simulink model "ResearchPaper4Fig9"  (R2015b)
settings: Solver=VariableStepAuto  StartTime=0.0  StopTime=10.0  RelTol=1e-3
libraries: xbsIndex_r4 x942, commfilt2 x1, commrandsrc3 x1, commdigbbndam3 x1
(part 2 of 6)

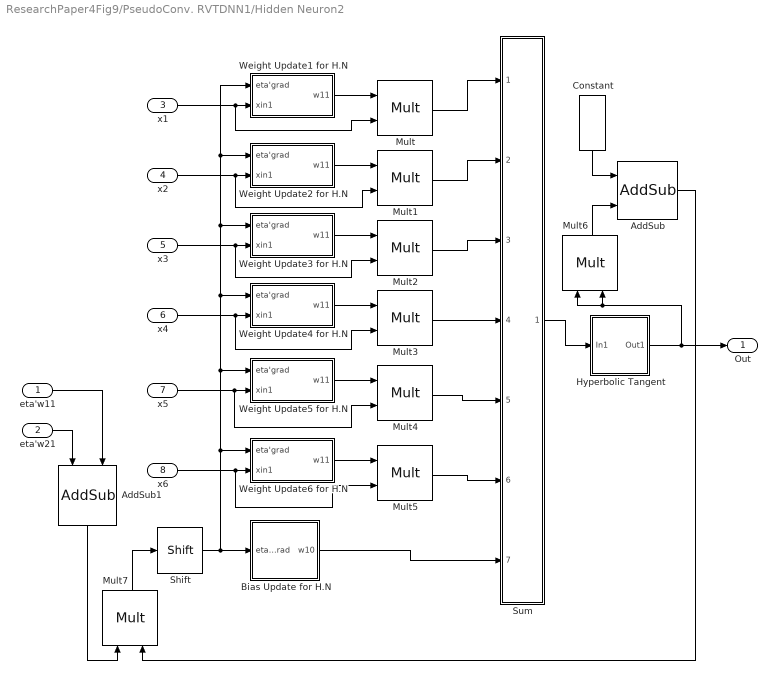
== system ResearchPaper4Fig9/PseudoConv. RVTDNN1/Hidden Neuron2 ==
  eta'w11 : Inport
  eta'w21 : Inport  Port=2
  x1 : Inport  Port=3
  x2 : Inport  Port=4
  x3 : Inport  Port=5
  x4 : Inport  Port=6
  x5 : Inport  Port=7
  x6 : Inport  Port=8
  AddSub : xbsIndex_r4/AddSub  mode=Subtraction  use_carryin=off  use_carryout=off  en=off  latency=0  precision=Full  arith_type=Unsigned  n_bits=16  bin_pt=14  quantization=Truncate  overflow=Wrap  use_behavioral_HDL=off  hw_selection=Fabric  pipelined=off  dbl_ovrd=off  block_type=addsub
  AddSub1 : xbsIndex_r4/AddSub  mode=Addition  use_carryin=off  use_carryout=off  en=off  latency=0  precision=Full  arith_type=Unsigned  n_bits=16  bin_pt=14  quantization=Truncate  overflow=Wrap  use_behavioral_HDL=off  hw_selection=Fabric  pipelined=off  dbl_ovrd=off  block_type=addsub
  Bias Update for H.N : Subsystem
  Constant : xbsIndex_r4/Constant  const=1.0  gui_display_data_type=Fixed-point  arith_type=Signed (2's comp)  n_bits=16  bin_pt=14  preci_type=Single  exp_width=8  frac_width=24  explicit_period=off  period=1  equ=P=C  opselect=C  inp2=PCIN>>17  opr=+  inp1=P  carry=CIN  dbl_ovrd=off  block_type=constant
  Hyperbolic Tangent : Subsystem
  Mult{,1..7} (8 alike) : xbsIndex_r4/Mult  precision=Full  arith_type="Signed  (2's comp)"  n_bits=16  bin_pt=14  quantization=Truncate  overflow=Wrap  en=off  latency=0  use_behavioral_HDL=off  opt=Speed  use_embedded=on  optimum_pipeline=off  pipeline=on  dbl_ovrd=off  use_rpm=on  placement_style=Triangular  block_type=mult
  Shift : xbsIndex_r4/Shift  shift_dir=Right  shift_bits=4  en=off  latency=0  precision=Full  arith_type="Signed  (2's comp)"  n_bits=16  bin_pt=14  quantization=Truncate  overflow=Wrap  dbl_ovrd=off  block_type=shift
  Sum : Subsystem
  Weight Update1 for H.N : Subsystem
  Weight Update2 for H.N : Subsystem
  Weight Update3 for H.N : Subsystem
  Weight Update4 for H.N : Subsystem
  Weight Update5 for H.N : Subsystem
  Weight Update6 for H.N : Subsystem
  Out : Outport
  wires:
  Mult7/1 -> Shift/1
  Constant/1 -> AddSub/1
  Shift/1 -> Weight Update6 for H.N/1(eta'grad), Weight Update5 for H.N/1(eta'grad), Weight Update4 for H.N/1(eta'grad), Weight Update3 for H.N/1(eta'grad), Weight Update2 for H.N/1(eta'grad), Weight Update1 for H.N/1(eta'grad), Bias Update for H.N/1(eta'grad)
  Mult6/1 -> AddSub/2
  eta'w11/1 -> AddSub1/2
  Hyperbolic Tangent/1(Out1) -> Out/1, Mult6/1, Mult6/2
  AddSub1/1 -> Mult7/1
  AddSub/1 -> Mult7/2
  eta'w21/1 -> AddSub1/1
  Weight Update5 for H.N/1(w11) -> Mult4/1
  x3/1 -> Weight Update3 for H.N/2(xin1), Mult2/2
  x5/1 -> Weight Update5 for H.N/2(xin1), Mult4/2
  Weight Update6 for H.N/1(w11) -> Mult5/1
  Weight Update4 for H.N/1(w11) -> Mult3/1
  x2/1 -> Weight Update2 for H.N/2(xin1), Mult1/2
  Weight Update1 for H.N/1(w11) -> Mult/1
  Weight Update2 for H.N/1(w11) -> Mult1/1
  Weight Update3 for H.N/1(w11) -> Mult2/1
  x1/1 -> Mult/2, Weight Update1 for H.N/2(xin1)
  x4/1 -> Weight Update4 for H.N/2(xin1), Mult3/2
  x6/1 -> Weight Update6 for H.N/2(xin1), Mult5/2
  Mult/1 -> Sum/1(In1)
  Mult1/1 -> Sum/2(In2)
  Mult2/1 -> Sum/3(In3)
  Mult3/1 -> Sum/4(In4)
  Mult4/1 -> Sum/5(In5)
  Mult5/1 -> Sum/6(In6)
  Bias Update for H.N/1(w10) -> Sum/7(In7)
  Sum/1(Out) -> Hyperbolic Tangent/1(In1)

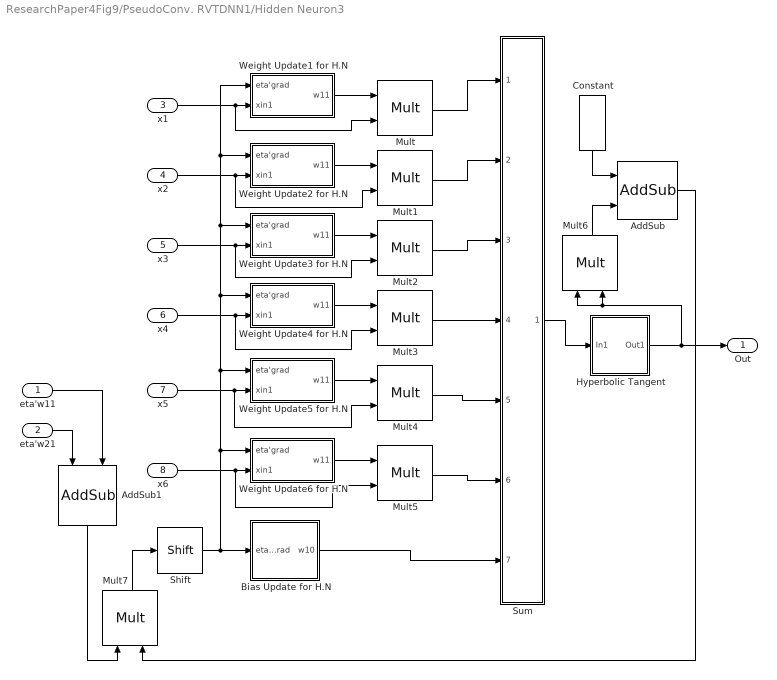
== system ResearchPaper4Fig9/PseudoConv. RVTDNN1/Hidden Neuron3 ==
  eta'w11 : Inport
  eta'w21 : Inport  Port=2
  x1 : Inport  Port=3
  x2 : Inport  Port=4
  x3 : Inport  Port=5
  x4 : Inport  Port=6
  x5 : Inport  Port=7
  x6 : Inport  Port=8
  AddSub : xbsIndex_r4/AddSub  mode=Subtraction  use_carryin=off  use_carryout=off  en=off  latency=0  precision=Full  arith_type=Unsigned  n_bits=16  bin_pt=14  quantization=Truncate  overflow=Wrap  use_behavioral_HDL=off  hw_selection=Fabric  pipelined=off  dbl_ovrd=off  block_type=addsub
  AddSub1 : xbsIndex_r4/AddSub  mode=Addition  use_carryin=off  use_carryout=off  en=off  latency=0  precision=Full  arith_type=Unsigned  n_bits=16  bin_pt=14  quantization=Truncate  overflow=Wrap  use_behavioral_HDL=off  hw_selection=Fabric  pipelined=off  dbl_ovrd=off  block_type=addsub
  Bias Update for H.N : Subsystem
  Constant : xbsIndex_r4/Constant  const=1.0  gui_display_data_type=Fixed-point  arith_type=Signed (2's comp)  n_bits=16  bin_pt=14  preci_type=Single  exp_width=8  frac_width=24  explicit_period=off  period=1  equ=P=C  opselect=C  inp2=PCIN>>17  opr=+  inp1=P  carry=CIN  dbl_ovrd=off  block_type=constant
  Hyperbolic Tangent : Subsystem
  Mult{,1..7} (8 alike) : xbsIndex_r4/Mult  precision=Full  arith_type="Signed  (2's comp)"  n_bits=16  bin_pt=14  quantization=Truncate  overflow=Wrap  en=off  latency=0  use_behavioral_HDL=off  opt=Speed  use_embedded=on  optimum_pipeline=off  pipeline=on  dbl_ovrd=off  use_rpm=on  placement_style=Triangular  block_type=mult
  Shift : xbsIndex_r4/Shift  shift_dir=Right  shift_bits=4  en=off  latency=0  precision=Full  arith_type="Signed  (2's comp)"  n_bits=16  bin_pt=14  quantization=Truncate  overflow=Wrap  dbl_ovrd=off  block_type=shift
  Sum : Subsystem
  Weight Update1 for H.N : Subsystem
  Weight Update2 for H.N : Subsystem
  Weight Update3 for H.N : Subsystem
  Weight Update4 for H.N : Subsystem
  Weight Update5 for H.N : Subsystem
  Weight Update6 for H.N : Subsystem
  Out : Outport
  wires:
  Mult7/1 -> Shift/1
  Constant/1 -> AddSub/1
  Shift/1 -> Weight Update6 for H.N/1(eta'grad), Weight Update5 for H.N/1(eta'grad), Weight Update4 for H.N/1(eta'grad), Weight Update3 for H.N/1(eta'grad), Weight Update2 for H.N/1(eta'grad), Weight Update1 for H.N/1(eta'grad), Bias Update for H.N/1(eta'grad)
  Mult6/1 -> AddSub/2
  eta'w11/1 -> AddSub1/2
  Hyperbolic Tangent/1(Out1) -> Out/1, Mult6/1, Mult6/2
  AddSub1/1 -> Mult7/1
  AddSub/1 -> Mult7/2
  eta'w21/1 -> AddSub1/1
  Weight Update5 for H.N/1(w11) -> Mult4/1
  x3/1 -> Weight Update3 for H.N/2(xin1), Mult2/2
  x5/1 -> Weight Update5 for H.N/2(xin1), Mult4/2
  Weight Update6 for H.N/1(w11) -> Mult5/1
  Weight Update4 for H.N/1(w11) -> Mult3/1
  x2/1 -> Weight Update2 for H.N/2(xin1), Mult1/2
  Weight Update1 for H.N/1(w11) -> Mult/1
  Weight Update2 for H.N/1(w11) -> Mult1/1
  Weight Update3 for H.N/1(w11) -> Mult2/1
  x1/1 -> Mult/2, Weight Update1 for H.N/2(xin1)
  x4/1 -> Weight Update4 for H.N/2(xin1), Mult3/2
  x6/1 -> Weight Update6 for H.N/2(xin1), Mult5/2
  Mult/1 -> Sum/1(In1)
  Mult1/1 -> Sum/2(In2)
  Mult2/1 -> Sum/3(In3)
  Mult3/1 -> Sum/4(In4)
  Mult4/1 -> Sum/5(In5)
  Mult5/1 -> Sum/6(In6)
  Bias Update for H.N/1(w10) -> Sum/7(In7)
  Sum/1(Out) -> Hyperbolic Tangent/1(In1)

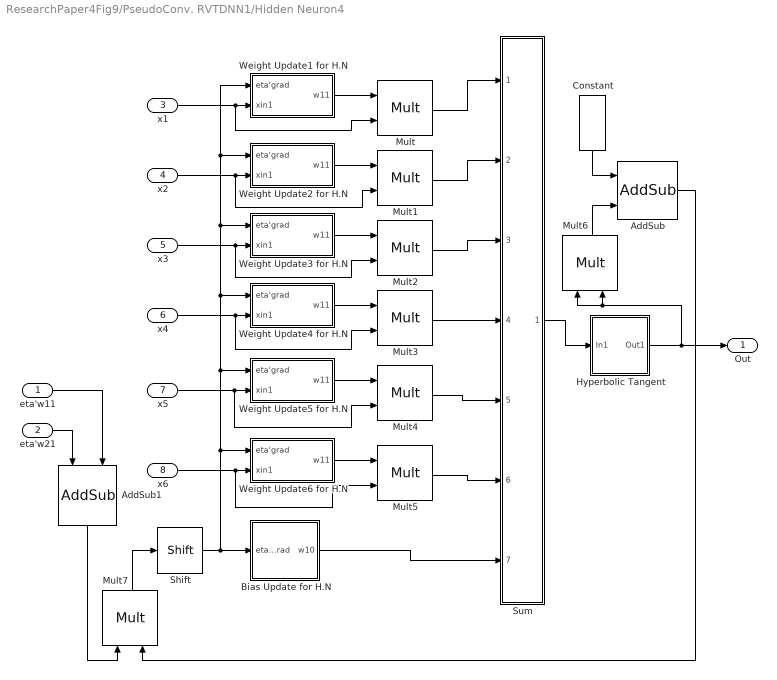
== system ResearchPaper4Fig9/PseudoConv. RVTDNN1/Hidden Neuron4 ==
  eta'w11 : Inport
  eta'w21 : Inport  Port=2
  x1 : Inport  Port=3
  x2 : Inport  Port=4
  x3 : Inport  Port=5
  x4 : Inport  Port=6
  x5 : Inport  Port=7
  x6 : Inport  Port=8
  AddSub : xbsIndex_r4/AddSub  mode=Subtraction  use_carryin=off  use_carryout=off  en=off  latency=0  precision=Full  arith_type=Unsigned  n_bits=16  bin_pt=14  quantization=Truncate  overflow=Wrap  use_behavioral_HDL=off  hw_selection=Fabric  pipelined=off  dbl_ovrd=off  block_type=addsub
  AddSub1 : xbsIndex_r4/AddSub  mode=Addition  use_carryin=off  use_carryout=off  en=off  latency=0  precision=Full  arith_type=Unsigned  n_bits=16  bin_pt=14  quantization=Truncate  overflow=Wrap  use_behavioral_HDL=off  hw_selection=Fabric  pipelined=off  dbl_ovrd=off  block_type=addsub
  Bias Update for H.N : Subsystem
  Constant : xbsIndex_r4/Constant  const=1.0  gui_display_data_type=Fixed-point  arith_type=Signed (2's comp)  n_bits=16  bin_pt=14  preci_type=Single  exp_width=8  frac_width=24  explicit_period=off  period=1  equ=P=C  opselect=C  inp2=PCIN>>17  opr=+  inp1=P  carry=CIN  dbl_ovrd=off  block_type=constant
  Hyperbolic Tangent : Subsystem
  Mult{,1..7} (8 alike) : xbsIndex_r4/Mult  precision=Full  arith_type="Signed  (2's comp)"  n_bits=16  bin_pt=14  quantization=Truncate  overflow=Wrap  en=off  latency=0  use_behavioral_HDL=off  opt=Speed  use_embedded=on  optimum_pipeline=off  pipeline=on  dbl_ovrd=off  use_rpm=on  placement_style=Triangular  block_type=mult
  Shift : xbsIndex_r4/Shift  shift_dir=Right  shift_bits=4  en=off  latency=0  precision=Full  arith_type="Signed  (2's comp)"  n_bits=16  bin_pt=14  quantization=Truncate  overflow=Wrap  dbl_ovrd=off  block_type=shift
  Sum : Subsystem
  Weight Update1 for H.N : Subsystem
  Weight Update2 for H.N : Subsystem
  Weight Update3 for H.N : Subsystem
  Weight Update4 for H.N : Subsystem
  Weight Update5 for H.N : Subsystem
  Weight Update6 for H.N : Subsystem
  Out : Outport
  wires:
  Mult7/1 -> Shift/1
  Constant/1 -> AddSub/1
  Shift/1 -> Weight Update6 for H.N/1(eta'grad), Weight Update5 for H.N/1(eta'grad), Weight Update4 for H.N/1(eta'grad), Weight Update3 for H.N/1(eta'grad), Weight Update2 for H.N/1(eta'grad), Weight Update1 for H.N/1(eta'grad), Bias Update for H.N/1(eta'grad)
  Mult6/1 -> AddSub/2
  eta'w11/1 -> AddSub1/2
  Hyperbolic Tangent/1(Out1) -> Out/1, Mult6/1, Mult6/2
  AddSub1/1 -> Mult7/1
  AddSub/1 -> Mult7/2
  eta'w21/1 -> AddSub1/1
  Weight Update5 for H.N/1(w11) -> Mult4/1
  x3/1 -> Weight Update3 for H.N/2(xin1), Mult2/2
  x5/1 -> Weight Update5 for H.N/2(xin1), Mult4/2
  Weight Update6 for H.N/1(w11) -> Mult5/1
  Weight Update4 for H.N/1(w11) -> Mult3/1
  x2/1 -> Weight Update2 for H.N/2(xin1), Mult1/2
  Weight Update1 for H.N/1(w11) -> Mult/1
  Weight Update2 for H.N/1(w11) -> Mult1/1
  Weight Update3 for H.N/1(w11) -> Mult2/1
  x1/1 -> Mult/2, Weight Update1 for H.N/2(xin1)
  x4/1 -> Weight Update4 for H.N/2(xin1), Mult3/2
  x6/1 -> Weight Update6 for H.N/2(xin1), Mult5/2
  Mult/1 -> Sum/1(In1)
  Mult1/1 -> Sum/2(In2)
  Mult2/1 -> Sum/3(In3)
  Mult3/1 -> Sum/4(In4)
  Mult4/1 -> Sum/5(In5)
  Mult5/1 -> Sum/6(In6)
  Bias Update for H.N/1(w10) -> Sum/7(In7)
  Sum/1(Out) -> Hyperbolic Tangent/1(In1)

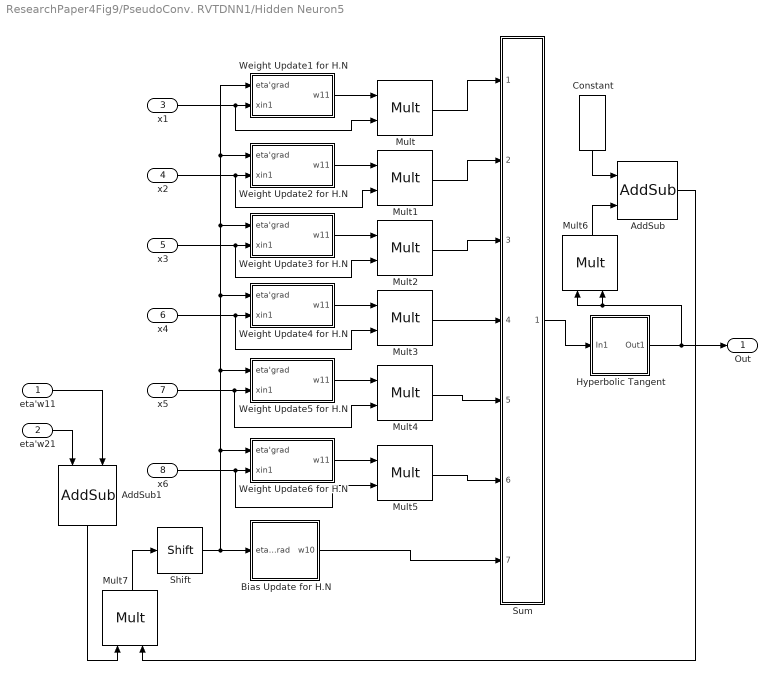
== system ResearchPaper4Fig9/PseudoConv. RVTDNN1/Hidden Neuron5 ==
  eta'w11 : Inport
  eta'w21 : Inport  Port=2
  x1 : Inport  Port=3
  x2 : Inport  Port=4
  x3 : Inport  Port=5
  x4 : Inport  Port=6
  x5 : Inport  Port=7
  x6 : Inport  Port=8
  AddSub : xbsIndex_r4/AddSub  mode=Subtraction  use_carryin=off  use_carryout=off  en=off  latency=0  precision=Full  arith_type=Unsigned  n_bits=16  bin_pt=14  quantization=Truncate  overflow=Wrap  use_behavioral_HDL=off  hw_selection=Fabric  pipelined=off  dbl_ovrd=off  block_type=addsub
  AddSub1 : xbsIndex_r4/AddSub  mode=Addition  use_carryin=off  use_carryout=off  en=off  latency=0  precision=Full  arith_type=Unsigned  n_bits=16  bin_pt=14  quantization=Truncate  overflow=Wrap  use_behavioral_HDL=off  hw_selection=Fabric  pipelined=off  dbl_ovrd=off  block_type=addsub
  Bias Update for H.N : Subsystem
  Constant : xbsIndex_r4/Constant  const=1.0  gui_display_data_type=Fixed-point  arith_type=Signed (2's comp)  n_bits=16  bin_pt=14  preci_type=Single  exp_width=8  frac_width=24  explicit_period=off  period=1  equ=P=C  opselect=C  inp2=PCIN>>17  opr=+  inp1=P  carry=CIN  dbl_ovrd=off  block_type=constant
  Hyperbolic Tangent : Subsystem
  Mult{,1..7} (8 alike) : xbsIndex_r4/Mult  precision=Full  arith_type="Signed  (2's comp)"  n_bits=16  bin_pt=14  quantization=Truncate  overflow=Wrap  en=off  latency=0  use_behavioral_HDL=off  opt=Speed  use_embedded=on  optimum_pipeline=off  pipeline=on  dbl_ovrd=off  use_rpm=on  placement_style=Triangular  block_type=mult
  Shift : xbsIndex_r4/Shift  shift_dir=Right  shift_bits=4  en=off  latency=0  precision=Full  arith_type="Signed  (2's comp)"  n_bits=16  bin_pt=14  quantization=Truncate  overflow=Wrap  dbl_ovrd=off  block_type=shift
  Sum : Subsystem
  Weight Update1 for H.N : Subsystem
  Weight Update2 for H.N : Subsystem
  Weight Update3 for H.N : Subsystem
  Weight Update4 for H.N : Subsystem
  Weight Update5 for H.N : Subsystem
  Weight Update6 for H.N : Subsystem
  Out : Outport
  wires:
  Mult7/1 -> Shift/1
  Constant/1 -> AddSub/1
  Shift/1 -> Weight Update6 for H.N/1(eta'grad), Weight Update5 for H.N/1(eta'grad), Weight Update4 for H.N/1(eta'grad), Weight Update3 for H.N/1(eta'grad), Weight Update2 for H.N/1(eta'grad), Weight Update1 for H.N/1(eta'grad), Bias Update for H.N/1(eta'grad)
  Mult6/1 -> AddSub/2
  eta'w11/1 -> AddSub1/2
  Hyperbolic Tangent/1(Out1) -> Out/1, Mult6/1, Mult6/2
  AddSub1/1 -> Mult7/1
  AddSub/1 -> Mult7/2
  eta'w21/1 -> AddSub1/1
  Weight Update5 for H.N/1(w11) -> Mult4/1
  x3/1 -> Weight Update3 for H.N/2(xin1), Mult2/2
  x5/1 -> Weight Update5 for H.N/2(xin1), Mult4/2
  Weight Update6 for H.N/1(w11) -> Mult5/1
  Weight Update4 for H.N/1(w11) -> Mult3/1
  x2/1 -> Weight Update2 for H.N/2(xin1), Mult1/2
  Weight Update1 for H.N/1(w11) -> Mult/1
  Weight Update2 for H.N/1(w11) -> Mult1/1
  Weight Update3 for H.N/1(w11) -> Mult2/1
  x1/1 -> Mult/2, Weight Update1 for H.N/2(xin1)
  x4/1 -> Weight Update4 for H.N/2(xin1), Mult3/2
  x6/1 -> Weight Update6 for H.N/2(xin1), Mult5/2
  Mult/1 -> Sum/1(In1)
  Mult1/1 -> Sum/2(In2)
  Mult2/1 -> Sum/3(In3)
  Mult3/1 -> Sum/4(In4)
  Mult4/1 -> Sum/5(In5)
  Mult5/1 -> Sum/6(In6)
  Bias Update for H.N/1(w10) -> Sum/7(In7)
  Sum/1(Out) -> Hyperbolic Tangent/1(In1)

== system ResearchPaper4Fig9/PseudoConv. RVTDNN1/Hidden Neuron6 ==
  eta'w11 : Inport
  eta'w21 : Inport  Port=2
  x1 : Inport  Port=3
  x2 : Inport  Port=4
  x3 : Inport  Port=5
  x4 : Inport  Port=6
  x5 : Inport  Port=7
  x6 : Inport  Port=8
  AddSub : xbsIndex_r4/AddSub  mode=Subtraction  use_carryin=off  use_carryout=off  en=off  latency=0  precision=Full  arith_type=Unsigned  n_bits=16  bin_pt=14  quantization=Truncate  overflow=Wrap  use_behavioral_HDL=off  hw_selection=Fabric  pipelined=off  dbl_ovrd=off  block_type=addsub
  AddSub1 : xbsIndex_r4/AddSub  mode=Addition  use_carryin=off  use_carryout=off  en=off  latency=0  precision=Full  arith_type=Unsigned  n_bits=16  bin_pt=14  quantization=Truncate  overflow=Wrap  use_behavioral_HDL=off  hw_selection=Fabric  pipelined=off  dbl_ovrd=off  block_type=addsub
  Bias Update for H.N : Subsystem
  Constant : xbsIndex_r4/Constant  const=1.0  gui_display_data_type=Fixed-point  arith_type=Signed (2's comp)  n_bits=16  bin_pt=14  preci_type=Single  exp_width=8  frac_width=24  explicit_period=off  period=1  equ=P=C  opselect=C  inp2=PCIN>>17  opr=+  inp1=P  carry=CIN  dbl_ovrd=off  block_type=constant
  Hyperbolic Tangent : Subsystem
  Mult{,1..7} (8 alike) : xbsIndex_r4/Mult  precision=Full  arith_type="Signed  (2's comp)"  n_bits=16  bin_pt=14  quantization=Truncate  overflow=Wrap  en=off  latency=0  use_behavioral_HDL=off  opt=Speed  use_embedded=on  optimum_pipeline=off  pipeline=on  dbl_ovrd=off  use_rpm=on  placement_style=Triangular  block_type=mult
  Shift : xbsIndex_r4/Shift  shift_dir=Right  shift_bits=4  en=off  latency=0  precision=Full  arith_type="Signed  (2's comp)"  n_bits=16  bin_pt=14  quantization=Truncate  overflow=Wrap  dbl_ovrd=off  block_type=shift
  Sum : Subsystem
  Weight Update1 for H.N : Subsystem
  Weight Update2 for H.N : Subsystem
  Weight Update3 for H.N : Subsystem
  Weight Update4 for H.N : Subsystem
  Weight Update5 for H.N : Subsystem
  Weight Update6 for H.N : Subsystem
  Out : Outport
  wires:
  Mult7/1 -> Shift/1
  Constant/1 -> AddSub/1
  Shift/1 -> Weight Update6 for H.N/1(eta'grad), Weight Update5 for H.N/1(eta'grad), Weight Update4 for H.N/1(eta'grad), Weight Update3 for H.N/1(eta'grad), Weight Update2 for H.N/1(eta'grad), Weight Update1 for H.N/1(eta'grad), Bias Update for H.N/1(eta'grad)
  Mult6/1 -> AddSub/2
  eta'w11/1 -> AddSub1/2
  Hyperbolic Tangent/1(Out1) -> Out/1, Mult6/1, Mult6/2
  AddSub1/1 -> Mult7/1
  AddSub/1 -> Mult7/2
  eta'w21/1 -> AddSub1/1
  Weight Update5 for H.N/1(w11) -> Mult4/1
  x3/1 -> Weight Update3 for H.N/2(xin1), Mult2/2
  x5/1 -> Weight Update5 for H.N/2(xin1), Mult4/2
  Weight Update6 for H.N/1(w11) -> Mult5/1
  Weight Update4 for H.N/1(w11) -> Mult3/1
  x2/1 -> Weight Update2 for H.N/2(xin1), Mult1/2
  Weight Update1 for H.N/1(w11) -> Mult/1
  Weight Update2 for H.N/1(w11) -> Mult1/1
  Weight Update3 for H.N/1(w11) -> Mult2/1
  x1/1 -> Mult/2, Weight Update1 for H.N/2(xin1)
  x4/1 -> Weight Update4 for H.N/2(xin1), Mult3/2
  x6/1 -> Weight Update6 for H.N/2(xin1), Mult5/2
  Mult/1 -> Sum/1(In1)
  Mult1/1 -> Sum/2(In2)
  Mult2/1 -> Sum/3(In3)
  Mult3/1 -> Sum/4(In4)
  Mult4/1 -> Sum/5(In5)
  Mult5/1 -> Sum/6(In6)
  Bias Update for H.N/1(w10) -> Sum/7(In7)
  Sum/1(Out) -> Hyperbolic Tangent/1(In1)

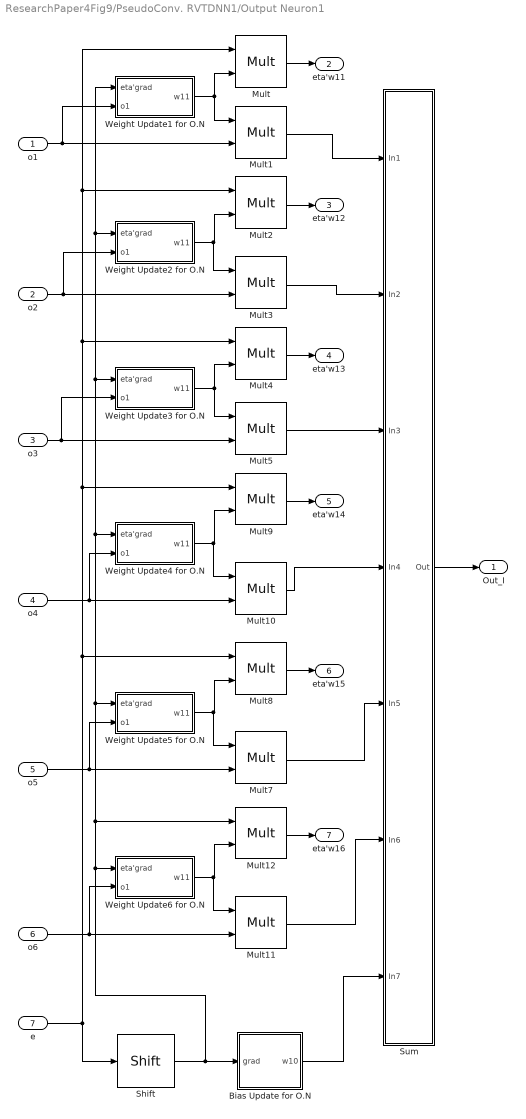
== system ResearchPaper4Fig9/PseudoConv. RVTDNN1/Output Neuron1 ==
  o1 : Inport
  o2 : Inport  Port=2
  o3 : Inport  Port=3
  o4 : Inport  Port=4
  o5 : Inport  Port=5
  o6 : Inport  Port=6
  e : Inport  Port=7
  Bias Update for O.N : Subsystem
  Mult{,1..5,7..12} (12 alike) : xbsIndex_r4/Mult  precision=Full  arith_type="Signed  (2's comp)"  n_bits=16  bin_pt=14  quantization=Truncate  overflow=Wrap  en=off  latency=0  use_behavioral_HDL=off  opt=Speed  use_embedded=on  optimum_pipeline=off  pipeline=on  dbl_ovrd=off  use_rpm=on  placement_style=Triangular  block_type=mult
  Shift : xbsIndex_r4/Shift  shift_dir=Right  shift_bits=4  en=off  latency=0  precision=Full  arith_type="Signed  (2's comp)"  n_bits=16  bin_pt=14  quantization=Truncate  overflow=Wrap  dbl_ovrd=off  block_type=shift
  Sum : Subsystem
  Weight Update1 for O.N : Subsystem
  Weight Update2 for O.N : Subsystem
  Weight Update3 for O.N : Subsystem
  Weight Update4 for O.N : Subsystem
  Weight Update5 for O.N : Subsystem
  Weight Update6 for O.N : Subsystem
  Out_I : Outport
  eta'w11 : Outport  Port=2
  eta'w12 : Outport  Port=3
  eta'w13 : Outport  Port=4
  eta'w14 : Outport  Port=5
  eta'w15 : Outport  Port=6
  eta'w16 : Outport  Port=7
  wires:
  o3/1 -> Weight Update3 for O.N/2(o1), Mult5/2
  o2/1 -> Weight Update2 for O.N/2(o1), Mult3/2
  o1/1 -> Weight Update1 for O.N/2(o1), Mult1/2
  o4/1 -> Weight Update4 for O.N/2(o1), Mult10/2
  Weight Update1 for O.N/1(w11) -> Mult1/1, Mult/2
  Weight Update2 for O.N/1(w11) -> Mult3/1, Mult2/2
  Weight Update3 for O.N/1(w11) -> Mult5/1, Mult4/2
  Weight Update4 for O.N/1(w11) -> Mult10/1, Mult9/2
  Mult/1 -> eta'w11/1
  Mult2/1 -> eta'w12/1
  Mult4/1 -> eta'w13/1
  Mult9/1 -> eta'w14/1
  Mult3/1 -> Sum/2(In2)
  Shift/1 -> Weight Update6 for O.N/1(eta'grad), Mult12/1, Weight Update5 for O.N/1(eta'grad), Weight Update4 for O.N/1(eta'grad), Weight Update3 for O.N/1(eta'grad), Weight Update2 for O.N/1(eta'grad), Weight Update1 for O.N/1(eta'grad), Bias Update for O.N/1(grad)
  e/1 -> Shift/1, Mult8/1, Mult4/1, Mult2/1, Mult/1, Mult9/1
  Sum/1(Out) -> Out_I/1
  o5/1 -> Weight Update5 for O.N/2(o1), Mult7/2
  Weight Update5 for O.N/1(w11) -> Mult7/1, Mult8/2
  Mult8/1 -> eta'w15/1
  o6/1 -> Weight Update6 for O.N/2(o1), Mult11/2
  Weight Update6 for O.N/1(w11) -> Mult11/1, Mult12/2
  Mult12/1 -> eta'w16/1
  Mult1/1 -> Sum/1(In1)
  Mult5/1 -> Sum/3(In3)
  Mult10/1 -> Sum/4(In4)
  Mult7/1 -> Sum/5(In5)
  Mult11/1 -> Sum/6(In6)
  Bias Update for O.N/1(w10) -> Sum/7(In7)

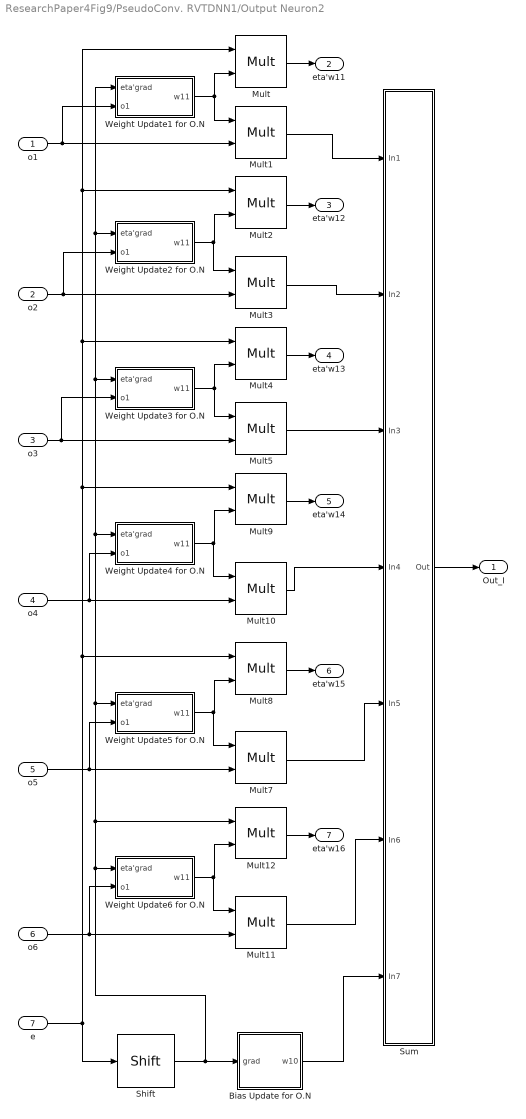
== system ResearchPaper4Fig9/PseudoConv. RVTDNN1/Output Neuron2 ==
  o1 : Inport
  o2 : Inport  Port=2
  o3 : Inport  Port=3
  o4 : Inport  Port=4
  o5 : Inport  Port=5
  o6 : Inport  Port=6
  e : Inport  Port=7
  Bias Update for O.N : Subsystem
  Mult{,1..5,7..12} (12 alike) : xbsIndex_r4/Mult  precision=Full  arith_type="Signed  (2's comp)"  n_bits=16  bin_pt=14  quantization=Truncate  overflow=Wrap  en=off  latency=0  use_behavioral_HDL=off  opt=Speed  use_embedded=on  optimum_pipeline=off  pipeline=on  dbl_ovrd=off  use_rpm=on  placement_style=Triangular  block_type=mult
  Shift : xbsIndex_r4/Shift  shift_dir=Right  shift_bits=4  en=off  latency=0  precision=Full  arith_type="Signed  (2's comp)"  n_bits=16  bin_pt=14  quantization=Truncate  overflow=Wrap  dbl_ovrd=off  block_type=shift
  Sum : Subsystem
  Weight Update1 for O.N : Subsystem
  Weight Update2 for O.N : Subsystem
  Weight Update3 for O.N : Subsystem
  Weight Update4 for O.N : Subsystem
  Weight Update5 for O.N : Subsystem
  Weight Update6 for O.N : Subsystem
  Out_I : Outport
  eta'w11 : Outport  Port=2
  eta'w12 : Outport  Port=3
  eta'w13 : Outport  Port=4
  eta'w14 : Outport  Port=5
  eta'w15 : Outport  Port=6
  eta'w16 : Outport  Port=7
  wires:
  o3/1 -> Weight Update3 for O.N/2(o1), Mult5/2
  o2/1 -> Weight Update2 for O.N/2(o1), Mult3/2
  o1/1 -> Weight Update1 for O.N/2(o1), Mult1/2
  o4/1 -> Weight Update4 for O.N/2(o1), Mult10/2
  Weight Update1 for O.N/1(w11) -> Mult1/1, Mult/2
  Weight Update2 for O.N/1(w11) -> Mult3/1, Mult2/2
  Weight Update3 for O.N/1(w11) -> Mult5/1, Mult4/2
  Weight Update4 for O.N/1(w11) -> Mult10/1, Mult9/2
  Mult/1 -> eta'w11/1
  Mult2/1 -> eta'w12/1
  Mult4/1 -> eta'w13/1
  Mult9/1 -> eta'w14/1
  Mult3/1 -> Sum/2(In2)
  Shift/1 -> Weight Update6 for O.N/1(eta'grad), Mult12/1, Weight Update5 for O.N/1(eta'grad), Weight Update4 for O.N/1(eta'grad), Weight Update3 for O.N/1(eta'grad), Weight Update2 for O.N/1(eta'grad), Weight Update1 for O.N/1(eta'grad), Bias Update for O.N/1(grad)
  e/1 -> Shift/1, Mult8/1, Mult4/1, Mult2/1, Mult/1, Mult9/1
  Sum/1(Out) -> Out_I/1
  o5/1 -> Weight Update5 for O.N/2(o1), Mult7/2
  Weight Update5 for O.N/1(w11) -> Mult7/1, Mult8/2
  Mult8/1 -> eta'w15/1
  o6/1 -> Weight Update6 for O.N/2(o1), Mult11/2
  Weight Update6 for O.N/1(w11) -> Mult11/1, Mult12/2
  Mult12/1 -> eta'w16/1
  Mult1/1 -> Sum/1(In1)
  Mult5/1 -> Sum/3(In3)
  Mult10/1 -> Sum/4(In4)
  Mult7/1 -> Sum/5(In5)
  Mult11/1 -> Sum/6(In6)
  Bias Update for O.N/1(w10) -> Sum/7(In7)

== system ResearchPaper4Fig9/PseudoConv. RVTDNN6/Hidden Neuron1 ==
  eta'w11 : Inport
  eta'w21 : Inport  Port=2
  x1 : Inport  Port=3
  x2 : Inport  Port=4
  x3 : Inport  Port=5
  x4 : Inport  Port=6
  x5 : Inport  Port=7
  x6 : Inport  Port=8
  AddSub : xbsIndex_r4/AddSub  mode=Subtraction  use_carryin=off  use_carryout=off  en=off  latency=0  precision=Full  arith_type=Unsigned  n_bits=16  bin_pt=14  quantization=Truncate  overflow=Wrap  use_behavioral_HDL=off  hw_selection=Fabric  pipelined=off  dbl_ovrd=off  block_type=addsub
  AddSub1 : xbsIndex_r4/AddSub  mode=Addition  use_carryin=off  use_carryout=off  en=off  latency=0  precision=Full  arith_type=Unsigned  n_bits=16  bin_pt=14  quantization=Truncate  overflow=Wrap  use_behavioral_HDL=off  hw_selection=Fabric  pipelined=off  dbl_ovrd=off  block_type=addsub
  Bias Update for H.N : Subsystem
  Constant : xbsIndex_r4/Constant  const=1.0  gui_display_data_type=Fixed-point  arith_type=Signed (2's comp)  n_bits=16  bin_pt=14  preci_type=Single  exp_width=8  frac_width=24  explicit_period=off  period=1  equ=P=C  opselect=C  inp2=PCIN>>17  opr=+  inp1=P  carry=CIN  dbl_ovrd=off  block_type=constant
  Hyperbolic Tangent : Subsystem
  Mult{,1..7} (8 alike) : xbsIndex_r4/Mult  precision=Full  arith_type="Signed  (2's comp)"  n_bits=16  bin_pt=14  quantization=Truncate  overflow=Wrap  en=off  latency=0  use_behavioral_HDL=off  opt=Speed  use_embedded=on  optimum_pipeline=off  pipeline=on  dbl_ovrd=off  use_rpm=on  placement_style=Triangular  block_type=mult
  Shift : xbsIndex_r4/Shift  shift_dir=Right  shift_bits=4  en=off  latency=0  precision=Full  arith_type="Signed  (2's comp)"  n_bits=16  bin_pt=14  quantization=Truncate  overflow=Wrap  dbl_ovrd=off  block_type=shift
  Sum : Subsystem
  Weight Update1 for H.N : Subsystem
  Weight Update2 for H.N : Subsystem
  Weight Update3 for H.N : Subsystem
  Weight Update4 for H.N : Subsystem
  Weight Update5 for H.N : Subsystem
  Weight Update6 for H.N : Subsystem
  Out : Outport
  wires:
  Mult7/1 -> Shift/1
  Constant/1 -> AddSub/1
  Shift/1 -> Weight Update6 for H.N/1(eta'grad), Weight Update5 for H.N/1(eta'grad), Weight Update4 for H.N/1(eta'grad), Weight Update3 for H.N/1(eta'grad), Weight Update2 for H.N/1(eta'grad), Weight Update1 for H.N/1(eta'grad), Bias Update for H.N/1(eta'grad)
  Mult6/1 -> AddSub/2
  eta'w11/1 -> AddSub1/2
  Hyperbolic Tangent/1(Out1) -> Out/1, Mult6/1, Mult6/2
  AddSub1/1 -> Mult7/1
  AddSub/1 -> Mult7/2
  eta'w21/1 -> AddSub1/1
  Weight Update5 for H.N/1(w11) -> Mult4/1
  x3/1 -> Weight Update3 for H.N/2(xin1), Mult2/2
  x5/1 -> Weight Update5 for H.N/2(xin1), Mult4/2
  Weight Update6 for H.N/1(w11) -> Mult5/1
  Weight Update4 for H.N/1(w11) -> Mult3/1
  x2/1 -> Weight Update2 for H.N/2(xin1), Mult1/2
  Weight Update1 for H.N/1(w11) -> Mult/1
  Weight Update2 for H.N/1(w11) -> Mult1/1
  Weight Update3 for H.N/1(w11) -> Mult2/1
  x1/1 -> Mult/2, Weight Update1 for H.N/2(xin1)
  x4/1 -> Weight Update4 for H.N/2(xin1), Mult3/2
  x6/1 -> Weight Update6 for H.N/2(xin1), Mult5/2
  Mult/1 -> Sum/1(In1)
  Mult1/1 -> Sum/2(In2)
  Mult2/1 -> Sum/3(In3)
  Mult3/1 -> Sum/4(In4)
  Mult4/1 -> Sum/5(In5)
  Mult5/1 -> Sum/6(In6)
  Bias Update for H.N/1(w10) -> Sum/7(In7)
  Sum/1(Out) -> Hyperbolic Tangent/1(In1)

== system ResearchPaper4Fig9/PseudoConv. RVTDNN6/Hidden Neuron2 ==
  eta'w11 : Inport
  eta'w21 : Inport  Port=2
  x1 : Inport  Port=3
  x2 : Inport  Port=4
  x3 : Inport  Port=5
  x4 : Inport  Port=6
  x5 : Inport  Port=7
  x6 : Inport  Port=8
  AddSub : xbsIndex_r4/AddSub  mode=Subtraction  use_carryin=off  use_carryout=off  en=off  latency=0  precision=Full  arith_type=Unsigned  n_bits=16  bin_pt=14  quantization=Truncate  overflow=Wrap  use_behavioral_HDL=off  hw_selection=Fabric  pipelined=off  dbl_ovrd=off  block_type=addsub
  AddSub1 : xbsIndex_r4/AddSub  mode=Addition  use_carryin=off  use_carryout=off  en=off  latency=0  precision=Full  arith_type=Unsigned  n_bits=16  bin_pt=14  quantization=Truncate  overflow=Wrap  use_behavioral_HDL=off  hw_selection=Fabric  pipelined=off  dbl_ovrd=off  block_type=addsub
  Bias Update for H.N : Subsystem
  Constant : xbsIndex_r4/Constant  const=1.0  gui_display_data_type=Fixed-point  arith_type=Signed (2's comp)  n_bits=16  bin_pt=14  preci_type=Single  exp_width=8  frac_width=24  explicit_period=off  period=1  equ=P=C  opselect=C  inp2=PCIN>>17  opr=+  inp1=P  carry=CIN  dbl_ovrd=off  block_type=constant
  Hyperbolic Tangent : Subsystem
  Mult{,1..7} (8 alike) : xbsIndex_r4/Mult  precision=Full  arith_type="Signed  (2's comp)"  n_bits=16  bin_pt=14  quantization=Truncate  overflow=Wrap  en=off  latency=0  use_behavioral_HDL=off  opt=Speed  use_embedded=on  optimum_pipeline=off  pipeline=on  dbl_ovrd=off  use_rpm=on  placement_style=Triangular  block_type=mult
  Shift : xbsIndex_r4/Shift  shift_dir=Right  shift_bits=4  en=off  latency=0  precision=Full  arith_type="Signed  (2's comp)"  n_bits=16  bin_pt=14  quantization=Truncate  overflow=Wrap  dbl_ovrd=off  block_type=shift
  Sum : Subsystem
  Weight Update1 for H.N : Subsystem
  Weight Update2 for H.N : Subsystem
  Weight Update3 for H.N : Subsystem
  Weight Update4 for H.N : Subsystem
  Weight Update5 for H.N : Subsystem
  Weight Update6 for H.N : Subsystem
  Out : Outport
  wires:
  Mult7/1 -> Shift/1
  Constant/1 -> AddSub/1
  Shift/1 -> Weight Update6 for H.N/1(eta'grad), Weight Update5 for H.N/1(eta'grad), Weight Update4 for H.N/1(eta'grad), Weight Update3 for H.N/1(eta'grad), Weight Update2 for H.N/1(eta'grad), Weight Update1 for H.N/1(eta'grad), Bias Update for H.N/1(eta'grad)
  Mult6/1 -> AddSub/2
  eta'w11/1 -> AddSub1/2
  Hyperbolic Tangent/1(Out1) -> Out/1, Mult6/1, Mult6/2
  AddSub1/1 -> Mult7/1
  AddSub/1 -> Mult7/2
  eta'w21/1 -> AddSub1/1
  Weight Update5 for H.N/1(w11) -> Mult4/1
  x3/1 -> Weight Update3 for H.N/2(xin1), Mult2/2
  x5/1 -> Weight Update5 for H.N/2(xin1), Mult4/2
  Weight Update6 for H.N/1(w11) -> Mult5/1
  Weight Update4 for H.N/1(w11) -> Mult3/1
  x2/1 -> Weight Update2 for H.N/2(xin1), Mult1/2
  Weight Update1 for H.N/1(w11) -> Mult/1
  Weight Update2 for H.N/1(w11) -> Mult1/1
  Weight Update3 for H.N/1(w11) -> Mult2/1
  x1/1 -> Mult/2, Weight Update1 for H.N/2(xin1)
  x4/1 -> Weight Update4 for H.N/2(xin1), Mult3/2
  x6/1 -> Weight Update6 for H.N/2(xin1), Mult5/2
  Mult/1 -> Sum/1(In1)
  Mult1/1 -> Sum/2(In2)
  Mult2/1 -> Sum/3(In3)
  Mult3/1 -> Sum/4(In4)
  Mult4/1 -> Sum/5(In5)
  Mult5/1 -> Sum/6(In6)
  Bias Update for H.N/1(w10) -> Sum/7(In7)
  Sum/1(Out) -> Hyperbolic Tangent/1(In1)

== system ResearchPaper4Fig9/PseudoConv. RVTDNN6/Hidden Neuron3 ==
  eta'w11 : Inport
  eta'w21 : Inport  Port=2
  x1 : Inport  Port=3
  x2 : Inport  Port=4
  x3 : Inport  Port=5
  x4 : Inport  Port=6
  x5 : Inport  Port=7
  x6 : Inport  Port=8
  AddSub : xbsIndex_r4/AddSub  mode=Subtraction  use_carryin=off  use_carryout=off  en=off  latency=0  precision=Full  arith_type=Unsigned  n_bits=16  bin_pt=14  quantization=Truncate  overflow=Wrap  use_behavioral_HDL=off  hw_selection=Fabric  pipelined=off  dbl_ovrd=off  block_type=addsub
  AddSub1 : xbsIndex_r4/AddSub  mode=Addition  use_carryin=off  use_carryout=off  en=off  latency=0  precision=Full  arith_type=Unsigned  n_bits=16  bin_pt=14  quantization=Truncate  overflow=Wrap  use_behavioral_HDL=off  hw_selection=Fabric  pipelined=off  dbl_ovrd=off  block_type=addsub
  Bias Update for H.N : Subsystem
  Constant : xbsIndex_r4/Constant  const=1.0  gui_display_data_type=Fixed-point  arith_type=Signed (2's comp)  n_bits=16  bin_pt=14  preci_type=Single  exp_width=8  frac_width=24  explicit_period=off  period=1  equ=P=C  opselect=C  inp2=PCIN>>17  opr=+  inp1=P  carry=CIN  dbl_ovrd=off  block_type=constant
  Hyperbolic Tangent : Subsystem
  Mult{,1..7} (8 alike) : xbsIndex_r4/Mult  precision=Full  arith_type="Signed  (2's comp)"  n_bits=16  bin_pt=14  quantization=Truncate  overflow=Wrap  en=off  latency=0  use_behavioral_HDL=off  opt=Speed  use_embedded=on  optimum_pipeline=off  pipeline=on  dbl_ovrd=off  use_rpm=on  placement_style=Triangular  block_type=mult
  Shift : xbsIndex_r4/Shift  shift_dir=Right  shift_bits=4  en=off  latency=0  precision=Full  arith_type="Signed  (2's comp)"  n_bits=16  bin_pt=14  quantization=Truncate  overflow=Wrap  dbl_ovrd=off  block_type=shift
  Sum : Subsystem
  Weight Update1 for H.N : Subsystem
  Weight Update2 for H.N : Subsystem
  Weight Update3 for H.N : Subsystem
  Weight Update4 for H.N : Subsystem
  Weight Update5 for H.N : Subsystem
  Weight Update6 for H.N : Subsystem
  Out : Outport
  wires:
  Mult7/1 -> Shift/1
  Constant/1 -> AddSub/1
  Shift/1 -> Weight Update6 for H.N/1(eta'grad), Weight Update5 for H.N/1(eta'grad), Weight Update4 for H.N/1(eta'grad), Weight Update3 for H.N/1(eta'grad), Weight Update2 for H.N/1(eta'grad), Weight Update1 for H.N/1(eta'grad), Bias Update for H.N/1(eta'grad)
  Mult6/1 -> AddSub/2
  eta'w11/1 -> AddSub1/2
  Hyperbolic Tangent/1(Out1) -> Out/1, Mult6/1, Mult6/2
  AddSub1/1 -> Mult7/1
  AddSub/1 -> Mult7/2
  eta'w21/1 -> AddSub1/1
  Weight Update5 for H.N/1(w11) -> Mult4/1
  x3/1 -> Weight Update3 for H.N/2(xin1), Mult2/2
  x5/1 -> Weight Update5 for H.N/2(xin1), Mult4/2
  Weight Update6 for H.N/1(w11) -> Mult5/1
  Weight Update4 for H.N/1(w11) -> Mult3/1
  x2/1 -> Weight Update2 for H.N/2(xin1), Mult1/2
  Weight Update1 for H.N/1(w11) -> Mult/1
  Weight Update2 for H.N/1(w11) -> Mult1/1
  Weight Update3 for H.N/1(w11) -> Mult2/1
  x1/1 -> Mult/2, Weight Update1 for H.N/2(xin1)
  x4/1 -> Weight Update4 for H.N/2(xin1), Mult3/2
  x6/1 -> Weight Update6 for H.N/2(xin1), Mult5/2
  Mult/1 -> Sum/1(In1)
  Mult1/1 -> Sum/2(In2)
  Mult2/1 -> Sum/3(In3)
  Mult3/1 -> Sum/4(In4)
  Mult4/1 -> Sum/5(In5)
  Mult5/1 -> Sum/6(In6)
  Bias Update for H.N/1(w10) -> Sum/7(In7)
  Sum/1(Out) -> Hyperbolic Tangent/1(In1)

== system ResearchPaper4Fig9/PseudoConv. RVTDNN6/Hidden Neuron4 ==
  eta'w11 : Inport
  eta'w21 : Inport  Port=2
  x1 : Inport  Port=3
  x2 : Inport  Port=4
  x3 : Inport  Port=5
  x4 : Inport  Port=6
  x5 : Inport  Port=7
  x6 : Inport  Port=8
  AddSub : xbsIndex_r4/AddSub  mode=Subtraction  use_carryin=off  use_carryout=off  en=off  latency=0  precision=Full  arith_type=Unsigned  n_bits=16  bin_pt=14  quantization=Truncate  overflow=Wrap  use_behavioral_HDL=off  hw_selection=Fabric  pipelined=off  dbl_ovrd=off  block_type=addsub
  AddSub1 : xbsIndex_r4/AddSub  mode=Addition  use_carryin=off  use_carryout=off  en=off  latency=0  precision=Full  arith_type=Unsigned  n_bits=16  bin_pt=14  quantization=Truncate  overflow=Wrap  use_behavioral_HDL=off  hw_selection=Fabric  pipelined=off  dbl_ovrd=off  block_type=addsub
  Bias Update for H.N : Subsystem
  Constant : xbsIndex_r4/Constant  const=1.0  gui_display_data_type=Fixed-point  arith_type=Signed (2's comp)  n_bits=16  bin_pt=14  preci_type=Single  exp_width=8  frac_width=24  explicit_period=off  period=1  equ=P=C  opselect=C  inp2=PCIN>>17  opr=+  inp1=P  carry=CIN  dbl_ovrd=off  block_type=constant
  Hyperbolic Tangent : Subsystem
  Mult{,1..7} (8 alike) : xbsIndex_r4/Mult  precision=Full  arith_type="Signed  (2's comp)"  n_bits=16  bin_pt=14  quantization=Truncate  overflow=Wrap  en=off  latency=0  use_behavioral_HDL=off  opt=Speed  use_embedded=on  optimum_pipeline=off  pipeline=on  dbl_ovrd=off  use_rpm=on  placement_style=Triangular  block_type=mult
  Shift : xbsIndex_r4/Shift  shift_dir=Right  shift_bits=4  en=off  latency=0  precision=Full  arith_type="Signed  (2's comp)"  n_bits=16  bin_pt=14  quantization=Truncate  overflow=Wrap  dbl_ovrd=off  block_type=shift
  Sum : Subsystem
  Weight Update1 for H.N : Subsystem
  Weight Update2 for H.N : Subsystem
  Weight Update3 for H.N : Subsystem
  Weight Update4 for H.N : Subsystem
  Weight Update5 for H.N : Subsystem
  Weight Update6 for H.N : Subsystem
  Out : Outport
  wires:
  Mult7/1 -> Shift/1
  Constant/1 -> AddSub/1
  Shift/1 -> Weight Update6 for H.N/1(eta'grad), Weight Update5 for H.N/1(eta'grad), Weight Update4 for H.N/1(eta'grad), Weight Update3 for H.N/1(eta'grad), Weight Update2 for H.N/1(eta'grad), Weight Update1 for H.N/1(eta'grad), Bias Update for H.N/1(eta'grad)
  Mult6/1 -> AddSub/2
  eta'w11/1 -> AddSub1/2
  Hyperbolic Tangent/1(Out1) -> Out/1, Mult6/1, Mult6/2
  AddSub1/1 -> Mult7/1
  AddSub/1 -> Mult7/2
  eta'w21/1 -> AddSub1/1
  Weight Update5 for H.N/1(w11) -> Mult4/1
  x3/1 -> Weight Update3 for H.N/2(xin1), Mult2/2
  x5/1 -> Weight Update5 for H.N/2(xin1), Mult4/2
  Weight Update6 for H.N/1(w11) -> Mult5/1
  Weight Update4 for H.N/1(w11) -> Mult3/1
  x2/1 -> Weight Update2 for H.N/2(xin1), Mult1/2
  Weight Update1 for H.N/1(w11) -> Mult/1
  Weight Update2 for H.N/1(w11) -> Mult1/1
  Weight Update3 for H.N/1(w11) -> Mult2/1
  x1/1 -> Mult/2, Weight Update1 for H.N/2(xin1)
  x4/1 -> Weight Update4 for H.N/2(xin1), Mult3/2
  x6/1 -> Weight Update6 for H.N/2(xin1), Mult5/2
  Mult/1 -> Sum/1(In1)
  Mult1/1 -> Sum/2(In2)
  Mult2/1 -> Sum/3(In3)
  Mult3/1 -> Sum/4(In4)
  Mult4/1 -> Sum/5(In5)
  Mult5/1 -> Sum/6(In6)
  Bias Update for H.N/1(w10) -> Sum/7(In7)
  Sum/1(Out) -> Hyperbolic Tangent/1(In1)

== system ResearchPaper4Fig9/PseudoConv. RVTDNN6/Hidden Neuron5 ==
  eta'w11 : Inport
  eta'w21 : Inport  Port=2
  x1 : Inport  Port=3
  x2 : Inport  Port=4
  x3 : Inport  Port=5
  x4 : Inport  Port=6
  x5 : Inport  Port=7
  x6 : Inport  Port=8
  AddSub : xbsIndex_r4/AddSub  mode=Subtraction  use_carryin=off  use_carryout=off  en=off  latency=0  precision=Full  arith_type=Unsigned  n_bits=16  bin_pt=14  quantization=Truncate  overflow=Wrap  use_behavioral_HDL=off  hw_selection=Fabric  pipelined=off  dbl_ovrd=off  block_type=addsub
  AddSub1 : xbsIndex_r4/AddSub  mode=Addition  use_carryin=off  use_carryout=off  en=off  latency=0  precision=Full  arith_type=Unsigned  n_bits=16  bin_pt=14  quantization=Truncate  overflow=Wrap  use_behavioral_HDL=off  hw_selection=Fabric  pipelined=off  dbl_ovrd=off  block_type=addsub
  Bias Update for H.N : Subsystem
  Constant : xbsIndex_r4/Constant  const=1.0  gui_display_data_type=Fixed-point  arith_type=Signed (2's comp)  n_bits=16  bin_pt=14  preci_type=Single  exp_width=8  frac_width=24  explicit_period=off  period=1  equ=P=C  opselect=C  inp2=PCIN>>17  opr=+  inp1=P  carry=CIN  dbl_ovrd=off  block_type=constant
  Hyperbolic Tangent : Subsystem
  Mult{,1..7} (8 alike) : xbsIndex_r4/Mult  precision=Full  arith_type="Signed  (2's comp)"  n_bits=16  bin_pt=14  quantization=Truncate  overflow=Wrap  en=off  latency=0  use_behavioral_HDL=off  opt=Speed  use_embedded=on  optimum_pipeline=off  pipeline=on  dbl_ovrd=off  use_rpm=on  placement_style=Triangular  block_type=mult
  Shift : xbsIndex_r4/Shift  shift_dir=Right  shift_bits=4  en=off  latency=0  precision=Full  arith_type="Signed  (2's comp)"  n_bits=16  bin_pt=14  quantization=Truncate  overflow=Wrap  dbl_ovrd=off  block_type=shift
  Sum : Subsystem
  Weight Update1 for H.N : Subsystem
  Weight Update2 for H.N : Subsystem
  Weight Update3 for H.N : Subsystem
  Weight Update4 for H.N : Subsystem
  Weight Update5 for H.N : Subsystem
  Weight Update6 for H.N : Subsystem
  Out : Outport
  wires:
  Mult7/1 -> Shift/1
  Constant/1 -> AddSub/1
  Shift/1 -> Weight Update6 for H.N/1(eta'grad), Weight Update5 for H.N/1(eta'grad), Weight Update4 for H.N/1(eta'grad), Weight Update3 for H.N/1(eta'grad), Weight Update2 for H.N/1(eta'grad), Weight Update1 for H.N/1(eta'grad), Bias Update for H.N/1(eta'grad)
  Mult6/1 -> AddSub/2
  eta'w11/1 -> AddSub1/2
  Hyperbolic Tangent/1(Out1) -> Out/1, Mult6/1, Mult6/2
  AddSub1/1 -> Mult7/1
  AddSub/1 -> Mult7/2
  eta'w21/1 -> AddSub1/1
  Weight Update5 for H.N/1(w11) -> Mult4/1
  x3/1 -> Weight Update3 for H.N/2(xin1), Mult2/2
  x5/1 -> Weight Update5 for H.N/2(xin1), Mult4/2
  Weight Update6 for H.N/1(w11) -> Mult5/1
  Weight Update4 for H.N/1(w11) -> Mult3/1
  x2/1 -> Weight Update2 for H.N/2(xin1), Mult1/2
  Weight Update1 for H.N/1(w11) -> Mult/1
  Weight Update2 for H.N/1(w11) -> Mult1/1
  Weight Update3 for H.N/1(w11) -> Mult2/1
  x1/1 -> Mult/2, Weight Update1 for H.N/2(xin1)
  x4/1 -> Weight Update4 for H.N/2(xin1), Mult3/2
  x6/1 -> Weight Update6 for H.N/2(xin1), Mult5/2
  Mult/1 -> Sum/1(In1)
  Mult1/1 -> Sum/2(In2)
  Mult2/1 -> Sum/3(In3)
  Mult3/1 -> Sum/4(In4)
  Mult4/1 -> Sum/5(In5)
  Mult5/1 -> Sum/6(In6)
  Bias Update for H.N/1(w10) -> Sum/7(In7)
  Sum/1(Out) -> Hyperbolic Tangent/1(In1)

== system ResearchPaper4Fig9/PseudoConv. RVTDNN6/Hidden Neuron6 ==
  eta'w11 : Inport
  eta'w21 : Inport  Port=2
  x1 : Inport  Port=3
  x2 : Inport  Port=4
  x3 : Inport  Port=5
  x4 : Inport  Port=6
  x5 : Inport  Port=7
  x6 : Inport  Port=8
  AddSub : xbsIndex_r4/AddSub  mode=Subtraction  use_carryin=off  use_carryout=off  en=off  latency=0  precision=Full  arith_type=Unsigned  n_bits=16  bin_pt=14  quantization=Truncate  overflow=Wrap  use_behavioral_HDL=off  hw_selection=Fabric  pipelined=off  dbl_ovrd=off  block_type=addsub
  AddSub1 : xbsIndex_r4/AddSub  mode=Addition  use_carryin=off  use_carryout=off  en=off  latency=0  precision=Full  arith_type=Unsigned  n_bits=16  bin_pt=14  quantization=Truncate  overflow=Wrap  use_behavioral_HDL=off  hw_selection=Fabric  pipelined=off  dbl_ovrd=off  block_type=addsub
  Bias Update for H.N : Subsystem
  Constant : xbsIndex_r4/Constant  const=1.0  gui_display_data_type=Fixed-point  arith_type=Signed (2's comp)  n_bits=16  bin_pt=14  preci_type=Single  exp_width=8  frac_width=24  explicit_period=off  period=1  equ=P=C  opselect=C  inp2=PCIN>>17  opr=+  inp1=P  carry=CIN  dbl_ovrd=off  block_type=constant
  Hyperbolic Tangent : Subsystem
  Mult{,1..7} (8 alike) : xbsIndex_r4/Mult  precision=Full  arith_type="Signed  (2's comp)"  n_bits=16  bin_pt=14  quantization=Truncate  overflow=Wrap  en=off  latency=0  use_behavioral_HDL=off  opt=Speed  use_embedded=on  optimum_pipeline=off  pipeline=on  dbl_ovrd=off  use_rpm=on  placement_style=Triangular  block_type=mult
  Shift : xbsIndex_r4/Shift  shift_dir=Right  shift_bits=4  en=off  latency=0  precision=Full  arith_type="Signed  (2's comp)"  n_bits=16  bin_pt=14  quantization=Truncate  overflow=Wrap  dbl_ovrd=off  block_type=shift
  Sum : Subsystem
  Weight Update1 for H.N : Subsystem
  Weight Update2 for H.N : Subsystem
  Weight Update3 for H.N : Subsystem
  Weight Update4 for H.N : Subsystem
  Weight Update5 for H.N : Subsystem
  Weight Update6 for H.N : Subsystem
  Out : Outport
  wires:
  Mult7/1 -> Shift/1
  Constant/1 -> AddSub/1
  Shift/1 -> Weight Update6 for H.N/1(eta'grad), Weight Update5 for H.N/1(eta'grad), Weight Update4 for H.N/1(eta'grad), Weight Update3 for H.N/1(eta'grad), Weight Update2 for H.N/1(eta'grad), Weight Update1 for H.N/1(eta'grad), Bias Update for H.N/1(eta'grad)
  Mult6/1 -> AddSub/2
  eta'w11/1 -> AddSub1/2
  Hyperbolic Tangent/1(Out1) -> Out/1, Mult6/1, Mult6/2
  AddSub1/1 -> Mult7/1
  AddSub/1 -> Mult7/2
  eta'w21/1 -> AddSub1/1
  Weight Update5 for H.N/1(w11) -> Mult4/1
  x3/1 -> Weight Update3 for H.N/2(xin1), Mult2/2
  x5/1 -> Weight Update5 for H.N/2(xin1), Mult4/2
  Weight Update6 for H.N/1(w11) -> Mult5/1
  Weight Update4 for H.N/1(w11) -> Mult3/1
  x2/1 -> Weight Update2 for H.N/2(xin1), Mult1/2
  Weight Update1 for H.N/1(w11) -> Mult/1
  Weight Update2 for H.N/1(w11) -> Mult1/1
  Weight Update3 for H.N/1(w11) -> Mult2/1
  x1/1 -> Mult/2, Weight Update1 for H.N/2(xin1)
  x4/1 -> Weight Update4 for H.N/2(xin1), Mult3/2
  x6/1 -> Weight Update6 for H.N/2(xin1), Mult5/2
  Mult/1 -> Sum/1(In1)
  Mult1/1 -> Sum/2(In2)
  Mult2/1 -> Sum/3(In3)
  Mult3/1 -> Sum/4(In4)
  Mult4/1 -> Sum/5(In5)
  Mult5/1 -> Sum/6(In6)
  Bias Update for H.N/1(w10) -> Sum/7(In7)
  Sum/1(Out) -> Hyperbolic Tangent/1(In1)

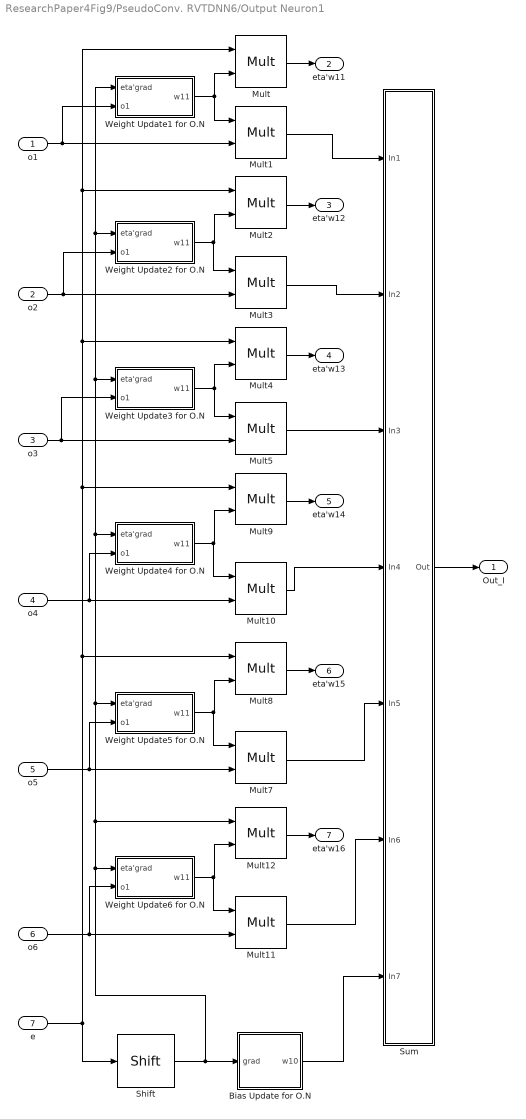
== system ResearchPaper4Fig9/PseudoConv. RVTDNN6/Output Neuron1 ==
  o1 : Inport
  o2 : Inport  Port=2
  o3 : Inport  Port=3
  o4 : Inport  Port=4
  o5 : Inport  Port=5
  o6 : Inport  Port=6
  e : Inport  Port=7
  Bias Update for O.N : Subsystem
  Mult{,1..5,7..12} (12 alike) : xbsIndex_r4/Mult  precision=Full  arith_type="Signed  (2's comp)"  n_bits=16  bin_pt=14  quantization=Truncate  overflow=Wrap  en=off  latency=0  use_behavioral_HDL=off  opt=Speed  use_embedded=on  optimum_pipeline=off  pipeline=on  dbl_ovrd=off  use_rpm=on  placement_style=Triangular  block_type=mult
  Shift : xbsIndex_r4/Shift  shift_dir=Right  shift_bits=4  en=off  latency=0  precision=Full  arith_type="Signed  (2's comp)"  n_bits=16  bin_pt=14  quantization=Truncate  overflow=Wrap  dbl_ovrd=off  block_type=shift
  Sum : Subsystem
  Weight Update1 for O.N : Subsystem
  Weight Update2 for O.N : Subsystem
  Weight Update3 for O.N : Subsystem
  Weight Update4 for O.N : Subsystem
  Weight Update5 for O.N : Subsystem
  Weight Update6 for O.N : Subsystem
  Out_I : Outport
  eta'w11 : Outport  Port=2
  eta'w12 : Outport  Port=3
  eta'w13 : Outport  Port=4
  eta'w14 : Outport  Port=5
  eta'w15 : Outport  Port=6
  eta'w16 : Outport  Port=7
  wires:
  o3/1 -> Weight Update3 for O.N/2(o1), Mult5/2
  o2/1 -> Weight Update2 for O.N/2(o1), Mult3/2
  o1/1 -> Weight Update1 for O.N/2(o1), Mult1/2
  o4/1 -> Weight Update4 for O.N/2(o1), Mult10/2
  Weight Update1 for O.N/1(w11) -> Mult1/1, Mult/2
  Weight Update2 for O.N/1(w11) -> Mult3/1, Mult2/2
  Weight Update3 for O.N/1(w11) -> Mult5/1, Mult4/2
  Weight Update4 for O.N/1(w11) -> Mult10/1, Mult9/2
  Mult/1 -> eta'w11/1
  Mult2/1 -> eta'w12/1
  Mult4/1 -> eta'w13/1
  Mult9/1 -> eta'w14/1
  Mult3/1 -> Sum/2(In2)
  Shift/1 -> Weight Update6 for O.N/1(eta'grad), Mult12/1, Weight Update5 for O.N/1(eta'grad), Weight Update4 for O.N/1(eta'grad), Weight Update3 for O.N/1(eta'grad), Weight Update2 for O.N/1(eta'grad), Weight Update1 for O.N/1(eta'grad), Bias Update for O.N/1(grad)
  e/1 -> Shift/1, Mult8/1, Mult4/1, Mult2/1, Mult/1, Mult9/1
  Sum/1(Out) -> Out_I/1
  o5/1 -> Weight Update5 for O.N/2(o1), Mult7/2
  Weight Update5 for O.N/1(w11) -> Mult7/1, Mult8/2
  Mult8/1 -> eta'w15/1
  o6/1 -> Weight Update6 for O.N/2(o1), Mult11/2
  Weight Update6 for O.N/1(w11) -> Mult11/1, Mult12/2
  Mult12/1 -> eta'w16/1
  Mult1/1 -> Sum/1(In1)
  Mult5/1 -> Sum/3(In3)
  Mult10/1 -> Sum/4(In4)
  Mult7/1 -> Sum/5(In5)
  Mult11/1 -> Sum/6(In6)
  Bias Update for O.N/1(w10) -> Sum/7(In7)

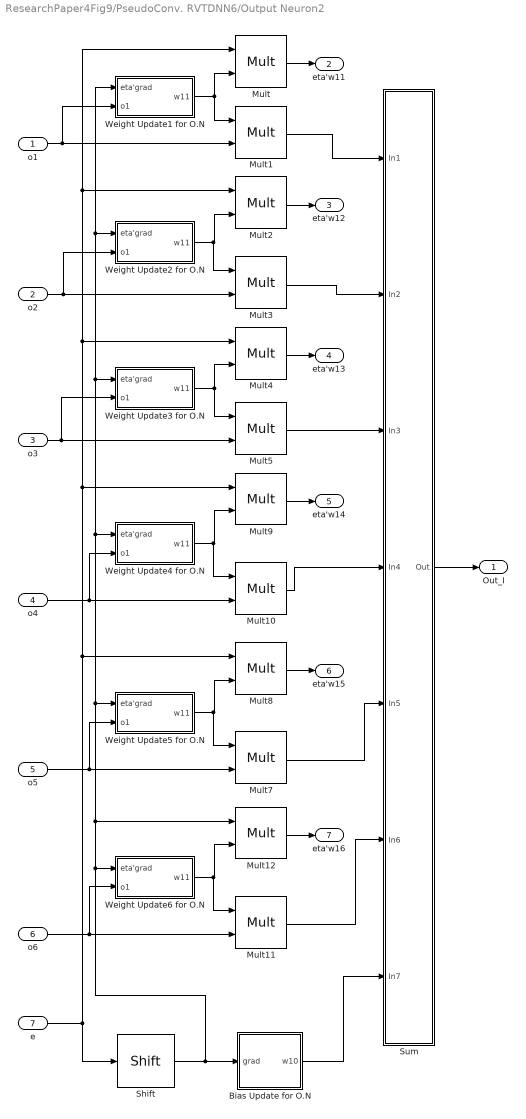
== system ResearchPaper4Fig9/PseudoConv. RVTDNN6/Output Neuron2 ==
  o1 : Inport
  o2 : Inport  Port=2
  o3 : Inport  Port=3
  o4 : Inport  Port=4
  o5 : Inport  Port=5
  o6 : Inport  Port=6
  e : Inport  Port=7
  Bias Update for O.N : Subsystem
  Mult{,1..5,7..12} (12 alike) : xbsIndex_r4/Mult  precision=Full  arith_type="Signed  (2's comp)"  n_bits=16  bin_pt=14  quantization=Truncate  overflow=Wrap  en=off  latency=0  use_behavioral_HDL=off  opt=Speed  use_embedded=on  optimum_pipeline=off  pipeline=on  dbl_ovrd=off  use_rpm=on  placement_style=Triangular  block_type=mult
  Shift : xbsIndex_r4/Shift  shift_dir=Right  shift_bits=4  en=off  latency=0  precision=Full  arith_type="Signed  (2's comp)"  n_bits=16  bin_pt=14  quantization=Truncate  overflow=Wrap  dbl_ovrd=off  block_type=shift
  Sum : Subsystem
  Weight Update1 for O.N : Subsystem
  Weight Update2 for O.N : Subsystem
  Weight Update3 for O.N : Subsystem
  Weight Update4 for O.N : Subsystem
  Weight Update5 for O.N : Subsystem
  Weight Update6 for O.N : Subsystem
  Out_I : Outport
  eta'w11 : Outport  Port=2
  eta'w12 : Outport  Port=3
  eta'w13 : Outport  Port=4
  eta'w14 : Outport  Port=5
  eta'w15 : Outport  Port=6
  eta'w16 : Outport  Port=7
  wires:
  o3/1 -> Weight Update3 for O.N/2(o1), Mult5/2
  o2/1 -> Weight Update2 for O.N/2(o1), Mult3/2
  o1/1 -> Weight Update1 for O.N/2(o1), Mult1/2
  o4/1 -> Weight Update4 for O.N/2(o1), Mult10/2
  Weight Update1 for O.N/1(w11) -> Mult1/1, Mult/2
  Weight Update2 for O.N/1(w11) -> Mult3/1, Mult2/2
  Weight Update3 for O.N/1(w11) -> Mult5/1, Mult4/2
  Weight Update4 for O.N/1(w11) -> Mult10/1, Mult9/2
  Mult/1 -> eta'w11/1
  Mult2/1 -> eta'w12/1
  Mult4/1 -> eta'w13/1
  Mult9/1 -> eta'w14/1
  Mult3/1 -> Sum/2(In2)
  Shift/1 -> Weight Update6 for O.N/1(eta'grad), Mult12/1, Weight Update5 for O.N/1(eta'grad), Weight Update4 for O.N/1(eta'grad), Weight Update3 for O.N/1(eta'grad), Weight Update2 for O.N/1(eta'grad), Weight Update1 for O.N/1(eta'grad), Bias Update for O.N/1(grad)
  e/1 -> Shift/1, Mult8/1, Mult4/1, Mult2/1, Mult/1, Mult9/1
  Sum/1(Out) -> Out_I/1
  o5/1 -> Weight Update5 for O.N/2(o1), Mult7/2
  Weight Update5 for O.N/1(w11) -> Mult7/1, Mult8/2
  Mult8/1 -> eta'w15/1
  o6/1 -> Weight Update6 for O.N/2(o1), Mult11/2
  Weight Update6 for O.N/1(w11) -> Mult11/1, Mult12/2
  Mult12/1 -> eta'w16/1
  Mult1/1 -> Sum/1(In1)
  Mult5/1 -> Sum/3(In3)
  Mult10/1 -> Sum/4(In4)
  Mult7/1 -> Sum/5(In5)
  Mult11/1 -> Sum/6(In6)
  Bias Update for O.N/1(w10) -> Sum/7(In7)

== system ResearchPaper4Fig9/PseudoConv. RVTDNN1/Hidden Neuron1/Bias Update for H.N ==
  eta'grad : Inport
  AddSub : xbsIndex_r4/AddSub  mode=Addition  use_carryin=off  use_carryout=off  en=off  latency=0  precision=Full  arith_type=Unsigned  n_bits=16  bin_pt=14  quantization=Truncate  overflow=Wrap  use_behavioral_HDL=off  hw_selection=Fabric  pipelined=off  dbl_ovrd=off  block_type=addsub
  Register : xbsIndex_r4/Register  init=0  rst=off  en=off  dbl_ovrd=off  block_type=register
  w10 : Outport
  wires:
  Register/1 -> w10/1, AddSub/2
  AddSub/1 -> Register/1
  eta'grad/1 -> AddSub/1

== system ResearchPaper4Fig9/PseudoConv. RVTDNN1/Hidden Neuron1/Hyperbolic Tangent ==
  In1 : Inport
  Constant : xbsIndex_r4/Constant  const=0.0  gui_display_data_type=Fixed-point  arith_type=Signed (2's comp)  n_bits=16  bin_pt=14  preci_type=Single  exp_width=8  frac_width=24  explicit_period=off  period=1  equ=P=C  opselect=C  inp2=PCIN>>17  opr=+  inp1=P  carry=CIN  dbl_ovrd=off  block_type=constant
  Delay : xbsIndex_r4/Delay  rst=off  infoeditControl=Selection of Reset will increase slice count due to use of real FFs and instead of SRLs  en=off  latency=1  reg_retiming=off  dbl_ovrd=off  block_type=delay
  Mux : xbsIndex_r4/Mux  inputs=2  en=off  latency=0  precision=Full  arith_type=Unsigned  n_bits=16  bin_pt=14  quantization=Truncate  overflow=Wrap  dbl_ovrd=off  block_type=mux
  Mux1 : xbsIndex_r4/Mux  inputs=2  en=off  latency=0  precision=Full  arith_type=Unsigned  n_bits=16  bin_pt=14  quantization=Truncate  overflow=Wrap  dbl_ovrd=off  block_type=mux
  Negate : xbsIndex_r4/Negate  precision=Full  arith_type=Unsigned  n_bits=16  bin_pt=14  quantization=Truncate  overflow=Wrap  en=off  latency=0  dbl_ovrd=off  block_type=negate
  Negate1 : xbsIndex_r4/Negate  precision=Full  arith_type=Unsigned  n_bits=16  bin_pt=14  quantization=Truncate  overflow=Wrap  en=off  latency=0  dbl_ovrd=off  block_type=negate
  ROM : xbsIndex_r4/ROM  depth=16  initVector=sin(pi*(0:15)/16)  distributed_mem=Distributed memory  rst=off  init_reg=0  en=off  latency=1  gui_display_data_type=Fixed-point  arith_type="Signed  (2's comp)"  n_bits=16  bin_pt=14  preci_type=Single  exp_width=8  frac_width=24  optimize=Area  use_rpm=on  dbl_ovrd=off  block_type=sprom
  Relational : xbsIndex_r4/Relational  mode=a>b  op_type=Bool  en=off  latency=0  dbl_ovrd=off  block_type=relational
  Shift : xbsIndex_r4/Shift  shift_dir=Left  shift_bits=13  en=off  latency=0  precision=Full  arith_type="Signed  (2's comp)"  n_bits=16  bin_pt=14  quantization=Truncate  overflow=Wrap  dbl_ovrd=off  block_type=shift
  Out1 : Outport
  wires:
  Relational/1 -> Delay/1, Mux/1
  Mux/1 -> Shift/1
  Mux1/1 -> Out1/1
  ROM/1 -> Negate1/1, Mux1/2
  Negate1/1 -> Mux1/3
  Constant/1 -> Relational/1
  In1/1 -> Negate/1, Relational/2, Mux/2
  Negate/1 -> Mux/3
  Shift/1 -> ROM/1
  Delay/1 -> Mux1/1
